simulink model "Project2P1a"  (R2017b)
settings: Solver=ode45  StartTime=0.0  StopTime=50.0  RelTol=1e-3  EnableMultiTasking=on
libraries: simulink x2
settings Model: Creator=Gopanraj  LastModifiedBy=Gopanraj
settings DataIOCC: LimitDataPoints=on  SaveFormat=Array  SignalLoggingSaveFormat=ModelDataLogs
settings OptimizationCC: ExpressionDepthLimit=2147483647  LifeSpan=inf
settings DebuggingCC: UnderspecifiedInitializationDetection=Classic  MergeDetectMultiDrivingBlocksExec=none  SolverPrmCheckMsg=warning  FcnCallInpInsideContextMsg=warning  StateNameClashWarn=warning  SFUnexpectedBacktrackingDiag=warning  SFNoUnconditionalDefaultTransitionDiag=warning  SFExecutionAtInitializationDiag=none
settings HardwareCC: ProdBitPerPointer=32  ProdBitPerSizeT=32  ProdBitPerPtrDiffT=32  ProdLargestAtomicFloat=None  ProdIntDivRoundTo=Undefined  ProdEndianess=Unspecified  ProdWordSize=32  ProdHWDeviceType=32-bit Generic
settings ModelReferenceCC: PropagateSignalLabelsOutOfModel=off
settings CodeAppCC: StateflowObjectComments=on
settings GRTTargetCC: TargetLangStandard=C89/C90 (ANSI)  GeneratePreprocessorConditionals=Disable all
settings ConfigComp: CovMetricSettings=dw  CovHtmlReporting=on  CovSaveCumulativeToWorkspaceVar=on  CovSaveSingleToWorkspaceVar=on  CovExternalEMLEnable=off

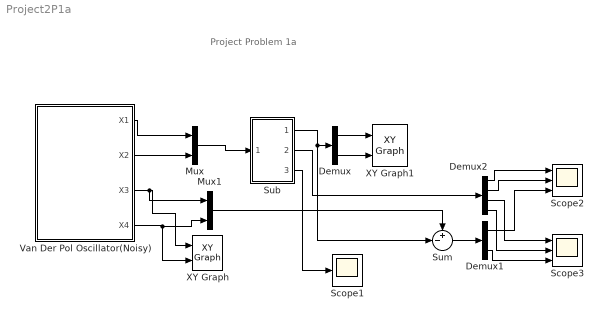
== system Project2P1a ==
  note: Project Problem 1a
  Demux : Demux  Outputs=2
  Demux1 : Demux  Outputs=2
  Demux2 : Demux
  Mux : Mux  Inputs=2
  Mux1 : Mux  Inputs=2
  Scope1 : Scope
  Scope2 : Scope  NumInputPorts=3
  Scope3 : Scope  NumInputPorts=3
  Sub : Subsystem
  Sum : Sum  Inputs=+-|
  Van Der Pol Oscillator(Noisy) : Subsystem
  XY Graph : simulink/Sinks/XY Graph  xmin=-4  xmax=4  ymin=-4  ymax=4  st=-1
  XY Graph1 : simulink/Sinks/XY Graph  xmin=-4  xmax=4  ymin=-4  ymax=4  st=-1
  wires:
  Van Der Pol Oscillator(Noisy)/1(X1) -> Mux/1
  Van Der Pol Oscillator(Noisy)/2(X2) -> Mux/2
  Mux/1 -> Sub/1(In1)
  Van Der Pol Oscillator(Noisy)/3(X3) -> Mux1/1, XY Graph/1
  Van Der Pol Oscillator(Noisy)/4(X4) -> Mux1/2, XY Graph/2
  Sub/1(Out1) -> Sum/2, Demux/1
  Demux/1 -> XY Graph1/1
  Demux/2 -> XY Graph1/2
  Sub/2(Out2) -> Demux2/1
  Sub/3(Out3) -> Scope1/1
  Sum/1 -> Demux1/1
  Demux2/1 -> Scope2/1
  Demux2/2 -> Scope2/2
  Demux1/1 -> Scope2/3
  Demux2/3 -> Scope3/1
  Demux2/4 -> Scope3/2
  Demux1/2 -> Scope3/3
  Mux1/1 -> Sum/1

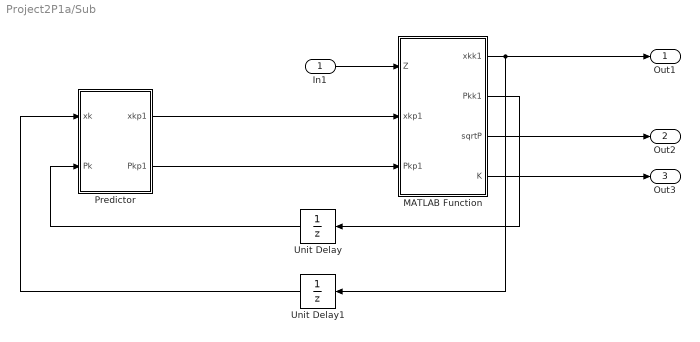
== system Project2P1a/Sub ==
  In1 : Inport
  MATLAB Function : MATLAB Function  TreatAsAtomicUnit=on
  Predictor : MATLAB Function  TreatAsAtomicUnit=on
  Unit Delay : UnitDelay  InitialCondition=eye(2)  SampleTime=-1
  Unit Delay1 : UnitDelay  InitialCondition=[0.1;0.1]  SampleTime=-1
  Out1 : Outport
  Out2 : Outport  Port=2
  Out3 : Outport  Port=3
  wires:
  MATLAB Function/1(xkk1) -> Unit Delay1/1, Out1/1
  MATLAB Function/2(Pkk1) -> Unit Delay/1
  Predictor/1(xkp1) -> MATLAB Function/2(xkp1)
  Predictor/2(Pkp1) -> MATLAB Function/3(Pkp1)
  Unit Delay1/1 -> Predictor/1(xk)
  In1/1 -> MATLAB Function/1(Z)
  MATLAB Function/3(sqrtP) -> Out2/1
  MATLAB Function/4(K) -> Out3/1
  Unit Delay/1 -> Predictor/2(Pk)

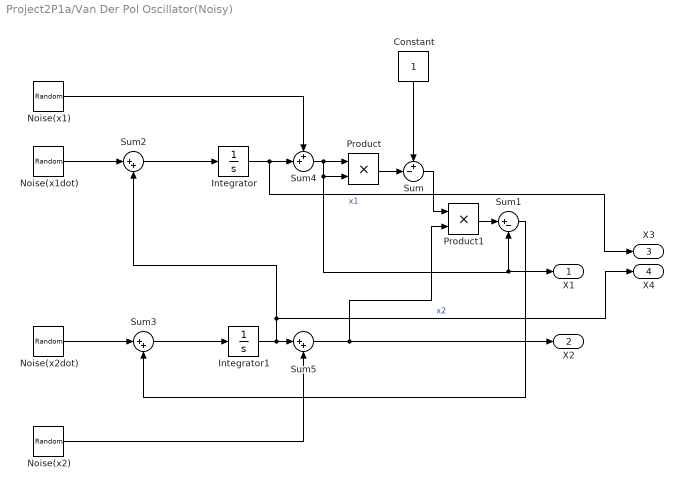
== system Project2P1a/Van Der Pol Oscillator(Noisy) ==
  Constant : Constant
  Integrator : Integrator  InitialCondition=0.1
  Integrator1 : Integrator  InitialCondition=0.1
  Noise(x1) : RandomNumber  Variance=0.015  Seed=73  SampleTime=0.1
  Noise(x1dot) : RandomNumber  Variance=0.2  Seed=43  SampleTime=0.1
  Noise(x2) : RandomNumber  Variance=0.025  Seed=87  SampleTime=0.1
  Noise(x2dot) : RandomNumber  Variance=0.1  Seed=57  SampleTime=0.1
  Product : Product
  Product1 : Product
  Sum : Sum  Inputs=+-|
  Sum1 : Sum  Inputs=|+-
  Sum2 : Sum  Inputs=|++
  Sum3 : Sum  Inputs=|++
  Sum4 : Sum  Inputs=++|
  Sum5 : Sum  Inputs=|++
  X1 : Outport
  X2 : Outport  Port=2
  X3 : Outport  Port=3
  X4 : Outport  Port=4
  wires:
  Sum3/1 -> Integrator1/1
  Sum2/1 -> Integrator/1
  Constant/1 -> Sum/1
  Sum/1 -> Product1/1
  Noise(x2)/1 -> Sum5/2
  Noise(x1dot)/1 -> Sum2/1
  Sum4/1 -> Sum1/2, X1/1, Product/2, Product/1
  Noise(x2dot)/1 -> Sum3/1
  Noise(x1)/1 -> Sum4/1
  Sum1/1 -> Sum3/2
  Product1/1 -> Sum1/1
  Integrator/1 -> X3/1, Sum4/2  "x1"
  Integrator1/1 -> X4/1, Sum2/2, Sum5/1  "x2"
  Sum5/1 -> X2/1, Product1/2
  Product/1 -> Sum/2

== matlab function Project2P1a/Sub/MATLAB Function ==
  data: Z input; xkk1 output; xkp1 input; Pkp1 input; Pkk1 output; sqrtP output; K output
function [xkk1, Pkk1,sqrtP,K] = corrector(Z,xkp1,Pkp1)

xkk1=zeros(2,1);
Pkk1=zeros(2);
sqrtP=zeros(4,1);

R=diag([0.015, 0.025]);

H=eye(2);
dh=eye(2);

K=Pkp1*dh'*inv(dh*Pkp1*(dh)'+R);
Pkk1=Pkp1- (K*(dh*Pkp1*(dh)'+R)*K');
xkk1=xkp1+K*(Z-H*xkp1);

P22=Pkk1(2,2);
sqrtP(4,1)=sqrt(abs(P22));
sqrtP(3,1)=-sqrt(abs(P22));
P11=Pkk1(1,1);
sqrtP(2,1)=sqrt(abs(P11));
sqrtP(1,1)=-sqrt(abs(P11));

end

== matlab function Project2P1a/Sub/Predictor ==
  data: xk input; xkp1 output; Pk input; Pkp1 output
function [xkp1, Pkp1] = predictor(xk, Pk)

xkp1=zeros(2,1);
Pkp1=zeros(2);

x1=xk(1);
x2=xk(2);
a =[0 1; -2*x1*x2-1 1-x1*x1];

Q = diag([2,1]);
T=0.1;
Ad=expm(a*T);

F=[-a Q;zeros(2,2) a'];
G=expm(F*T);
GLr=G(3:4,3:4);
Gur=G(1:2,3:4);
Qd=GLr'*Gur;

xkp1=Ad*xk;
Pkp1=Ad*Pk*Ad'+Qd;

end
